simulink model "derivador_puro"  (R2017b)
settings: Solver=VariableStepAuto  StartTime=0.0  StopTime=5  RelTol=1e-3
settings Model: Creator=fernandopassold  LastModifiedBy=fernandopassold

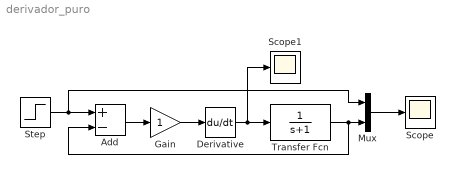
== system derivador_puro ==
  Add : Sum  Inputs=+-
  Derivative : Derivative
  Gain : Gain
  Mux : Mux  Inputs=2
  Scope : Scope
  Scope1 : Scope
  Step : Step  SampleTime=0
  Transfer Fcn : TransferFcn  Denominator=[1 1]
  wires:
  Step/1 -> Mux/1, Add/1
  Add/1 -> Gain/1
  Gain/1 -> Derivative/1
  Derivative/1 -> Scope1/1, Transfer Fcn/1
  Mux/1 -> Scope/1
  Transfer Fcn/1 -> Add/2, Mux/2
